simulink subsystem "Torue_Eq"  (R2022b)
settings: Solver=VariableStepAuto  StartTime=0.0  StopTime=10.0  RelTol=1e-3
model mask{P=P}
  mask prompts: P "No. of Pole Pairs"
settings Model: Creator=MAAM  LastModifiedBy=MAAM

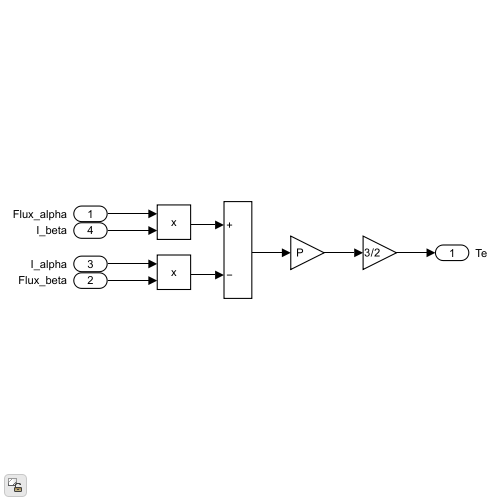
[thumbnail: Simulink's stored preview of the top-level diagram]
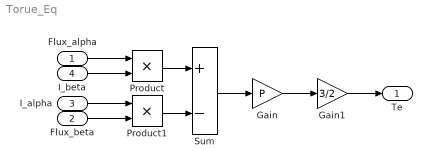
== system Torue_Eq ==
  Flux_alpha : Inport
  Flux_beta : Inport  Port=2
  I_alpha : Inport  Port=3
  I_beta : Inport  Port=4
  Gain : Gain  Gain=P
  Gain1 : Gain  Gain=3/2
  Product : Product
  Product1 : Product
  Sum : Sum  Inputs=+-
  Te : Outport
  wires:
  Flux_alpha/1 -> Product/1
  I_beta/1 -> Product/2
  I_alpha/1 -> Product1/1
  Flux_beta/1 -> Product1/2
  Product/1 -> Sum/1
  Product1/1 -> Sum/2
  Sum/1 -> Gain/1
  Gain/1 -> Gain1/1
  Gain1/1 -> Te/1
